simulink model "untitled"  (R2022b)
settings: Solver=FixedStepDiscrete  StartTime=0.0  StopTime=inf  FixedStep=1  MaxStep=1  RelTol=1e-3
(part 2 of 2)

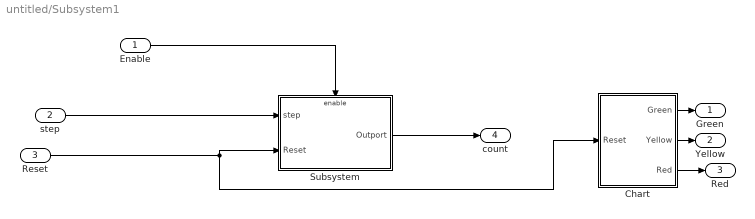
== system untitled/Subsystem1 ==
  Enable : Inport
  step : Inport  Port=2
  Reset : Inport  Port=3
  Chart : Stateflow chart  TreatAsAtomicUnit=on
  Subsystem : Subsystem
  Green : Outport
  Yellow : Outport  Port=2
  Red : Outport  Port=3
  count : Outport  Port=4
  wires:
  Reset/1 -> Chart/1(Reset), Subsystem/2(Reset)
  step/1 -> Subsystem/1(step)
  Chart/1(Green) -> Green/1
  Enable/1 -> Subsystem/Enable
  Chart/2(Yellow) -> Yellow/1
  Subsystem/1(Outport) -> count/1
  Chart/3(Red) -> Red/1

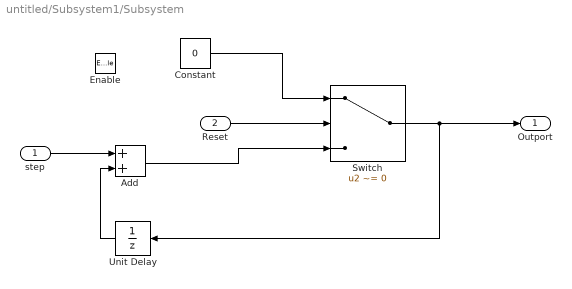
== system untitled/Subsystem1/Subsystem ==
  step : Inport
  Reset : Inport  Port=2
  Enable : EnablePort
  Add : Sum
  Constant : Constant  Value=0
  Switch : Switch  Criteria=u2 ~= 0  SaturateOnIntegerOverflow=off  InputSameDT=off
  Unit Delay : UnitDelay  SampleTime=-1  HasFrameUpgradeWarning=on
      settings: AttributesFormatString=InitialCondition=0
  Outport : Outport
  wires:
  Add/1 -> Switch/3
  Unit Delay/1 -> Add/2
  step/1 -> Add/1
  Reset/1 -> Switch/2
  Constant/1 -> Switch/1
  Switch/1 -> Unit Delay/1, Outport/1

== stateflow chart untitled/Subsystem1/Chart ==
  state LED_Yellow
    entry:
    Yellow=1;
    exit:
    Yellow=0;
  state LED_Red
    entry:
    Red=1;
    exit:
    Red=0;
  state LED_Green
    entry:
    Green=1;
    exit:
    Green=0;
  state on
    entry:
    Red=0;
    Yellow=0;
    Green=0;
  (default) -> on
  LED_Red -> LED_Yellow [order 1] : after(5,sec)
  LED_Yellow -> LED_Green [order 1] : after(4,sec)
  on -> LED_Red : [Reset==0]
  LED_Red -> on [order 2] : [Reset==1]
  LED_Green -> (junction 7) [order 1] : after(20,sec)
  LED_Green -> (junction 114) [order 2] : [Reset==1]
  (junction 11) -> LED_Red
  LED_Yellow -> (junction 112) [order 2] : [Reset==1]
  (junction 113) -> on
  (junction 7) -> (junction 11)
  (junction 114) -> (junction 112)
  (junction 112) -> (junction 113)
  data: Green output; Yellow output; Red output; Reset input
